simulink model "watermelon_simscape2"  (R2017b)
settings: Solver=ode14x  StartTime=0.0  StopTime=10000  FixedStep=.1  RelTol=1e-3
libraries: fl_lib x5, nesl_utility x3, aerolibconvert2 x2
settings Model: Creator=Harrison  LastModifiedBy=Harrison
settings DataIOCC: SaveFormat=Array

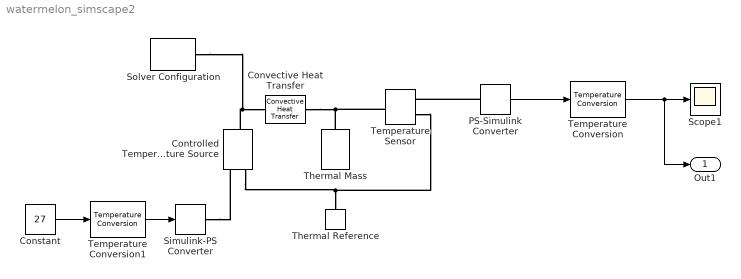
== system watermelon_simscape2 ==
  Constant : Constant  Value=27
  Controlled Temperature Source : fl_lib/Thermal/Thermal Sources/Controlled Temperature Source
      settings: SourceProductName=Simscape
  Convective Heat Transfer : fl_lib/Thermal/Thermal Elements/Convective Heat Transfer  area=4*pi*.2^2 m^2  heat_tr_coeff=15 W/(m^2 * K)  T_specify=on  T_priority=None  T=22 K  T_nominal_specify=off  T_nominal_unit=K  T_nominal_value=1  Q_specify=off  Q_priority=None  Q=0 W  Q_nominal_specify=off  Q_nominal_unit=W  Q_nominal_value=1
  PS-Simulink Converter : nesl_utility/PS-Simulink Converter  PhysicalDomain=network_engine_domain  SubClassName=ps_output  LeftPortType=input  RightPortType=output  PseudoPeriodic=off  Frequencies=[]  Unit=K  AffineConversion=on
  Scope1 : Scope
  Simulink-PS Converter : nesl_utility/Simulink-PS Converter  PhysicalDomain=network_engine_domain  SubClassName=ps_input  LeftPortType=input  RightPortType=output  PseudoPeriodic=off  Frequencies=[]  NoiseDistribution=none  NoiseParameters=[]  Unit=K  AffineConversion=on  FilteringAndDerivatives=provide  SimscapeFilterOrder=1  InputFilterTimeConstant=0.001  UdotUserProvided=0
  Solver Configuration : nesl_utility/Solver Configuration  PhysicalDomain=network_engine_domain  SubClassName=solver  LeftPortType=input  RightPortType=generic  Accelerate=off  Tones=[]  Harmonics=[]  SimulateNoise=off  Profile=off  UseLocalSampling=off  EnableSwitchedLinearOptims=on  FrequencyDomain=off  UseCCode=off  RelTol=0.001  AbsTol=1e-06  MinStep=1e-09  ToWorkspace=off  RevertToSquareIcSolve=off  NumHomotopyIterations=100  PhasorMode=off  PhasorModeNumHarmonics=1  DoDC=off  ResidualTolerance=1e-09  UseLocalSolver=off  LocalSolverChoice=NE_BACKWARD_EULER_ADVANCER  LocalSolverSampleTime=0.001  DoFixedCost=off  MaxNonlinIter=3  MaxModeIter=2  LinearAlgebra=Sparse  DelaysMemoryBudget=1024  AutomaticFiltering=on  FilteringTimeConstant=0.001
  Temperature Conversion : aerolibconvert2/Temperature Conversion  IU=K  OU=C
      settings: SourceProductName=Aerospace Blockset  SourceProductBaseCode=AE
  Temperature Conversion1 : aerolibconvert2/Temperature Conversion  IU=C  OU=K
      settings: SourceProductName=Aerospace Blockset  SourceProductBaseCode=AE
  Temperature Sensor : fl_lib/Thermal/Thermal Sensors/Temperature Sensor
  Thermal Mass : fl_lib/Thermal/Thermal Elements/Thermal Mass  mass=(4/3)*pi*(.2^3)*(120) kg  sp_heat=4200 J/kg/K  T_specify=on  T_priority=High  T=278 K  T_nominal_specify=off  T_nominal_unit=K  T_nominal_value=1  Q_specify=off  Q_priority=None  Q=0 W  Q_nominal_specify=off  Q_nominal_unit=W  Q_nominal_value=1
  Thermal Reference : fl_lib/Thermal/Thermal Elements/Thermal Reference
  Out1 : Outport
  wires:
  PS-Simulink Converter/1 -> Temperature Conversion/1
  Constant/1 -> Temperature Conversion1/1
  Temperature Conversion/1 -> Out1/1, Scope1/1
  Temperature Conversion1/1 -> Simulink-PS Converter/1
  connections:
  Thermal Mass/LConn1 -- Convective Heat Transfer/RConn1 -- Temperature Sensor/LConn1
  Simulink-PS Converter/RConn1 -- Controlled Temperature Source/RConn1
  Controlled Temperature Source/LConn1 -- Solver Configuration/RConn1 -- Convective Heat Transfer/LConn1
  PS-Simulink Converter/LConn1 -- Temperature Sensor/RConn2
  Controlled Temperature Source/RConn2 -- Temperature Sensor/RConn1 -- Thermal Reference/LConn1
